simulink model "sensor_test_MIL"  (R2022b)
settings: Solver=FixedStepDiscrete  StartTime=0.0  StopTime=30.0  RelTol=1e-3
InitFcn:
  | mbd_s32k_consistency_checks(bdroot(gcs));
undefined symbols (not defined in the file): LQFP
libraries: mbd_s32k1xx_ec_toolbox x4, hdlsllib x3, aerolibanimutils x1
settings Model: Creator=termi  LastModifiedBy=termi
settings DataIOCC: ExternalInput=off  InitialState=off  SaveOutput=off  SignalLogging=off  SaveTime=off
settings OptimizationCC: DefaultParameterBehavior=Inlined  EnhancedBackFolding=on  PassReuseOutputArgsAs=Individual arguments  ZeroExternalMemoryAtStartup=off  ZeroInternalMemoryAtStartup=off  OptimizeBlockOrder=speed  DifferentSizesBufferReuse=on  OptimizationCustomize=off  EfficientTunableParamExpr=on
settings DebuggingCC: InheritedTsInSrcMsg=none  SingleTaskRateTransMsg=error  ParameterTunabilityLossMsg=error  UnconnectedInputMsg=error  UnconnectedOutputMsg=error  UnconnectedLineMsg=error  UnknownTsInhSupMsg=error
settings HardwareCC: ProdBitPerPointer=32  ProdBitPerSizeT=32  ProdBitPerPtrDiffT=32  ProdLargestAtomicInteger=Long  ProdLargestAtomicFloat=Double  ProdWordSize=32  ProdHWDeviceType=ARM Compatible->ARM Cortex
settings SFSimCC: MATLABDynamicMemAlloc=off
settings RTWCC: Description=Model Based Design Toolbox S32K1xx Code Generation Target  SystemTargetFile=mbd_s32k.tlc  MakeCommand=mbd_s32k_make_rtw COPY_MDLREF_INCLUDES=0  TemplateMakefile=mbd_s32k.tmf
settings CodeAppCC: ForceParamTrailComments=on  IgnoreCustomStorageClasses=off  OperatorAnnotations=on  SimulinkDataObjDesc=on  SFDataObjDesc=on  InsertBlockDesc=on
settings STFCustomTargetCC: TargetLangStandard=C99 (ISO)  MultiwordLength=256  GenerateSampleERTMain=on  CombineOutputUpdateFcns=on  ERTCustomFileBanners=on  SupportContinuousTime=off  SupportNonInlinedSFcns=off  RemoveResetFunc=on  MATLABClassNameForMDSCustomization=Simulink.SoftwareTarget.ERTCustomization  SystemTargetFile=mbd_s32k.tlc
settings ERTTargetCC: TargetLangStandard=C99 (ISO)  GenerateSampleERTMain=on  ParMdlRefBuildCompliant=off  CompOptLevelCompliant=off  ConcurrentExecutionCompliant=off  ModelStepFunctionPrototypeControlCompliant=off  CPPClassGenCompliant=off  UseToolchainInfoCompliant=off  InlinedParameterPlacement=NonHierarchical  ERTSrcFileBannerTemplate=mbd_ert_code_template.cgt  ERTHdrFileBannerTemplate=mbd_ert_code_template.cgt  ERTDataSrcFileTemplate=mbd_ert_code_template.cgt  ERTDataHdrFileTemplate=mbd_ert_code_template.cgt  ERTCustomFileTemplate=example_file_process.tlc

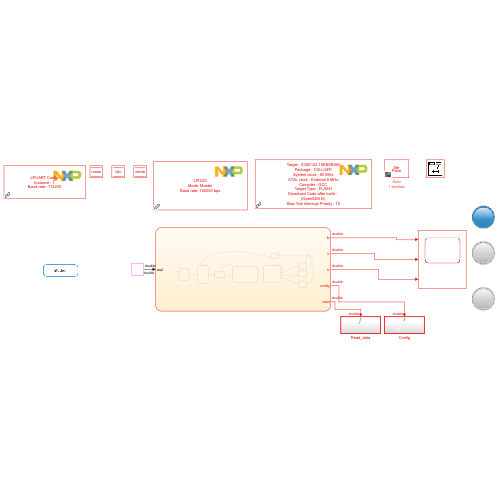
[thumbnail: Simulink's stored preview of the top-level diagram]
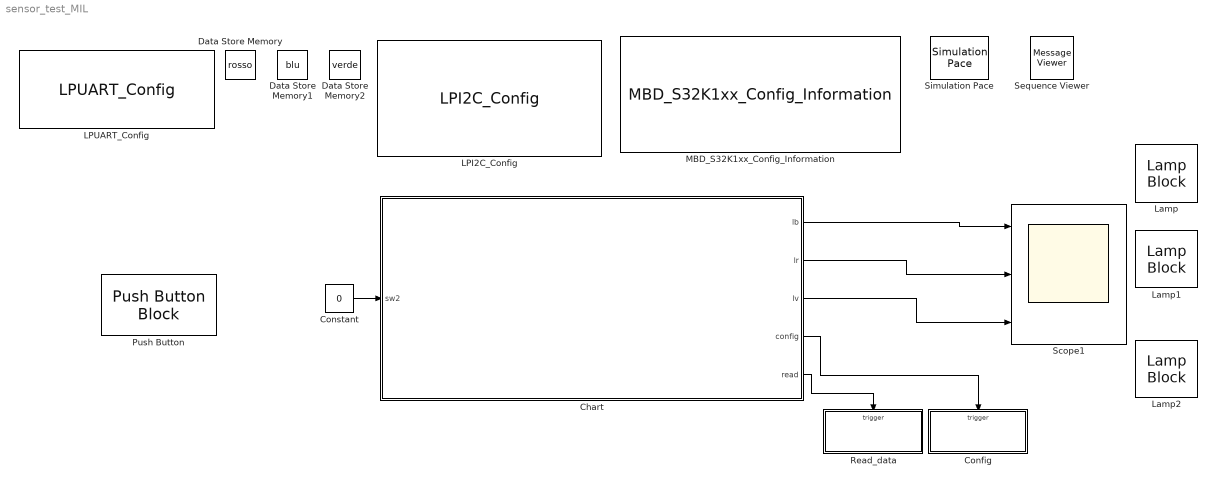
== system sensor_test_MIL ==
  Chart : Stateflow chart  TreatAsAtomicUnit=on
  Config : Subsystem  TreatAsAtomicUnit=on
  Constant : Constant  Value=0
  Data Store Memory : DataStoreMemory  DataStoreName=rosso  WriteAfterWriteMsg=warning  ShowAdditionalParam=off  OutDataTypeStr=uint16
  Data Store Memory1 : DataStoreMemory  DataStoreName=blu  WriteAfterWriteMsg=warning  ShowAdditionalParam=off  OutDataTypeStr=uint16
  Data Store Memory2 : DataStoreMemory  DataStoreName=verde  WriteAfterWriteMsg=warning  ShowAdditionalParam=off  OutDataTypeStr=uint16
  LPI2C_Config : mbd_s32k1xx_ec_toolbox/Communication Blocks/I2C Blocks/LPI2C_Config  Priority=1  instance=0  mode=Master  opmode=Standard (up to 100 kbit/s)  bdr=100000  addr=1  is10bitaddr=off  status=off  sda=PTA2: [LPI2C0_SDA | LPI2C Data I/O]  scl=PTA3: [LPI2C0_SCL | LPI2C Clock I/O]
  LPUART_Config : mbd_s32k1xx_ec_toolbox/Communication Blocks/UART Blocks/LPUART_Config  instance=1  baudrate=115200  custom_baudrate=1000000  databits=8  parity=None  sbns=1  bothedge=rising edge  rxinv=off  txinv=off  show_adv_opts=on  brk13=10 - 13 bit times  lbkde=10 - 13 bit times  rx=PTC6: [LPUART1_RX | Receive]  tx=PTC7: [LPUART1_TX | Transmit]
  Lamp : LampBlock  LabelPosition=Hide
  Lamp1 : LampBlock  LabelPosition=Hide
  Lamp2 : LampBlock  LabelPosition=Hide
  MBD_S32K1xx_Config_Information : mbd_s32k1xx_ec_toolbox/MBD_S32K1xx_Config_Information  Priority=1  mbdt_ver=0  disp_str=|  config_params=[]  mcu_target_name=S32K142  mcu_target_package=100-LQFP  mcu_target_sram_size=16KB  mcu_system_clock_freq=80  mcu_xtal_freq=External 8  mcu_steptick_timer=LPIT Channel 0  mcu_steptick_prio=15  ds_import_enable=on  target_compiler=GCC  target_memory=FLASH  gcc_target_compile_opts=-mthumb -mfloat-abi=hard -mfpu=fpv4-sp-d16 -O1 -g -gstrict-dwarf  gcc_target_assemble_opts=-mthumb -mfloat-abi=hard -mfpu=fpv4-sp-d16 -g  gcc_target_link_opts=-mthumb -mfloat-abi=hard -mfpu=fpv4-sp-d16  gcc_target_default_lcf=on  gcc_target_user_lcf=S32K142_16_flash.ld  ghs_target_compile_opts=-cpu=cortexm4f -thumb -fpu=vfpv4_d16 -fsingle -Ogeneral -Wundef -Wimplicit-int -Wshadow -Wtrigraphs --no_commons --gnu_asm -gnu99 -gdwarf-2 -G  ghs_target_assemble_opts=-cpu=cortexm4f -fpu=vfpv4_d16  ghs_target_link_opts=-cpu=cortexm4f -thumb -fpu=vfpv4_d16  ghs_target_default_lcf=on  ghs_target_user_lcf=S32K142_16_flash.ld  iar_target_compile_opts=--cpu=Cortex-M4F --thumb --fpu=VFPv4_sp -Ol -e --debug --dlib_config normal  iar_target_assemble_opts=--cpu Cortex-M4F --thumb --fpu VFPv4_sp  iar_target_link_opts=--no_exceptions --vfe --inline  iar_target_default_lcf=on  iar_target_user_lcf=S32K142_16_flash.icf  pil_download_enable=off  rbl_download_enable=on  rbl_start_delay=5000  rbl_download_interface=OpenSDA  rbl_restart_request=off  rbl_com_port=Custom  rbl_com_port_custom=COM3  pil_download_rate=115200  pil_download_rate_custom=115200  pil_opensda_drive=Custom  pil_opensda_drive_custom=D  jtag_interface=OpenSDA Embedded Debug  jlink_default_path=on  jlink_user_path=C:\Program Files\SEGGER\JLink\  pil_uart_instance=1  pil_uart_rx=PTC6: [LPUART1_RX | Receive]  pil_uart_tx=PTC7: [LPUART1_TX | Transmit]  FTM_PWM_PcrCheckEnDis=on  FTM_Input_Edge_Inputs_PcrCheckEnDis=on  FTM_Dual_Edge_Inputs_PcrCheckEnDis=on  FTM_Quadrature_Inputs_PcrCheckEnDis=on  FTM_Hall_Sensor_Inputs_PcrCheckEnDis=on  LPTMR_PcrCheckEnDis=on  PIT_PcrCheckEnDis=on  RTC_PcrCheckEnDis=on  FlexCAN_PcrCheckEnDis=on  LIN_PcrCheckEnDis=on  FlexIO_PcrCheckEnDis=on  LPI2C_PcrCheckEnDis=on  LPSPI_PcrCheckEnDis=on  LPUART_PcrCheckEnDis=on  CMP_PcrCheckEnDis=on  GPIO_OutputPcrCheckEnDis=on  GPIO_InputPcrCheckEnDis=on  SBC_PcrCheckEnDis=on  BMS_PcrCheckEnDis=on  AMMCLIB_PcrCheckEnDis=on  FM_PcrCheckEnDis=on  Profile_PcrCheckEnDis=on  ConfigParams_PcrCheckEnDis=on  ModelRef_PcrCheckEnDis=on  PDB0_PcrCheckEnDis=on  CSEc_PcrCheckEnDis=on  eDMA_PcrCheckEnDis=on  FLASH_PcrCheckEnDis=on  ADC_PcrCheckEnDis=on  WDOG_PcrCheckEnDis=on
      | Target : S32K144-64KB_SRAM
      | Package : 100-pin
      | System clock : 80 MHz
      | XTAL clock : External 8 MHz
      | Compiler : IAR
      | Target Type : FLASH
      | Download Code after build : off
      | Step Tick Interrupt Priority : 15
  Push Button : PushButtonBlock  OffValue=0.000000
  Read_data : Subsystem  TreatAsAtomicUnit=on
  Scope1 : Scope  NumInputPorts=3
  Sequence Viewer : MessageViewer
  Simulation Pace : aerolibanimutils/Simulation Pace  SimulationPace=1  SleepMode=Auto  OutputPaceError=off  SampleTime=1/10
  wires:
  Chart/1(lb) -> Scope1/1
  Chart/4(config) -> Config/Trigger
  Chart/3(lv) -> Scope1/3
  Chart/2(lr) -> Scope1/2
  Chart/5(read) -> Read_data/Trigger
  Constant/1 -> Chart/1(sw2)

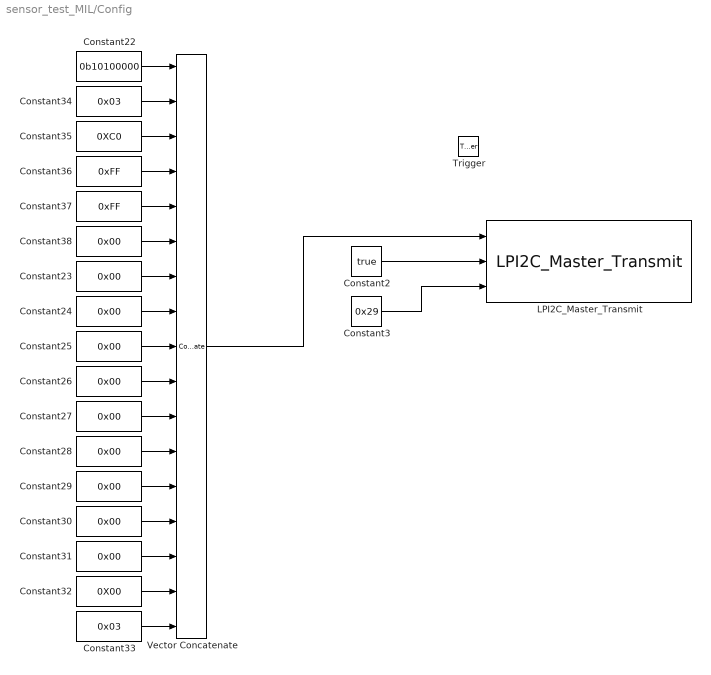
== system sensor_test_MIL/Config ==
  Trigger : TriggerPort  VariantControl=(inherit)  PortDimensions=1
  Constant2 : Constant  Value=true  OutDataTypeStr=boolean
  Constant22 : Constant  Value=0b10100000
  Constant{23..31,38} (10 alike) : Constant  Value=0x00
  Constant3 : Constant  Value=0x29  OutDataTypeStr=uint16
  Constant32 : Constant  Value=0X00
  Constant33 : Constant  Value=0x03
  Constant34 : Constant  Value=0x03
  Constant35 : Constant  Value=0XC0
  Constant36 : Constant  Value=0xFF
  Constant37 : Constant  Value=0xFF
  LPI2C_Master_Transmit : mbd_s32k1xx_ec_toolbox/Communication Blocks/I2C Blocks/LPI2C_Master_Transmit  Priority=1  instance=0  xfermode=Blocking  Timeout=710  is10bit=off  status=off
  Vector Concatenate : Concatenate  NumInputs=17
  wires:
  Constant27/1 -> Vector Concatenate/11
  Constant31/1 -> Vector Concatenate/15
  Constant33/1 -> Vector Concatenate/17
  Constant32/1 -> Vector Concatenate/16
  Constant30/1 -> Vector Concatenate/14
  Vector Concatenate/1 -> LPI2C_Master_Transmit/1
  Constant23/1 -> Vector Concatenate/7
  Constant28/1 -> Vector Concatenate/12
  Constant29/1 -> Vector Concatenate/13
  Constant3/1 -> LPI2C_Master_Transmit/3
  Constant36/1 -> Vector Concatenate/4
  Constant34/1 -> Vector Concatenate/2
  Constant24/1 -> Vector Concatenate/8
  Constant35/1 -> Vector Concatenate/3
  Constant26/1 -> Vector Concatenate/10
  Constant38/1 -> Vector Concatenate/6
  Constant25/1 -> Vector Concatenate/9
  Constant37/1 -> Vector Concatenate/5
  Constant2/1 -> LPI2C_Master_Transmit/2
  Constant22/1 -> Vector Concatenate/1

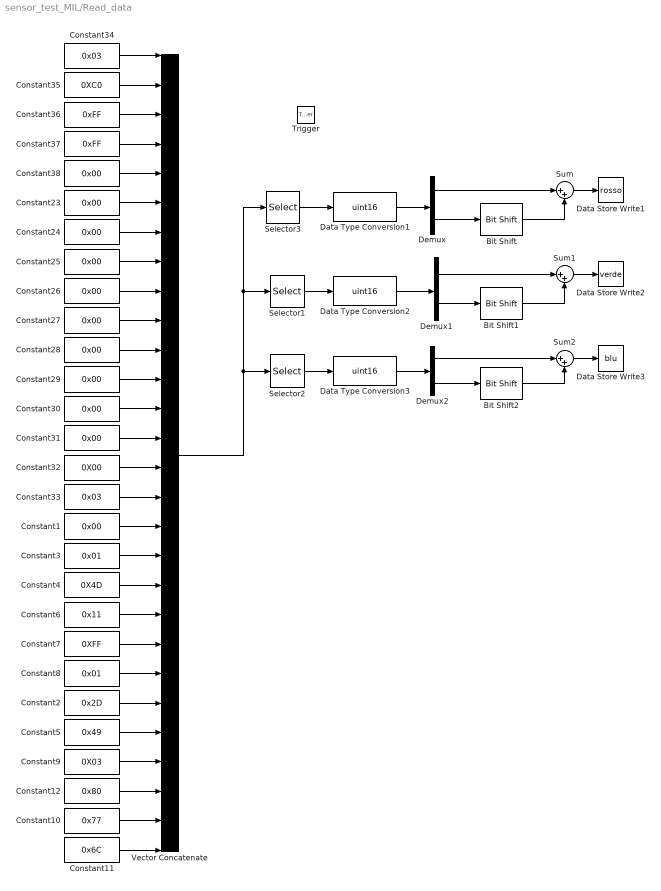
== system sensor_test_MIL/Read_data ==
  Trigger : TriggerPort  VariantControl=(inherit)  PortDimensions=1
  Bit Shift : hdlsllib/Logic and Bit Operations/Bit Shift  mode=Shift Left Logical  N=8
  Bit Shift1 : hdlsllib/Logic and Bit Operations/Bit Shift  mode=Shift Left Logical  N=8
  Bit Shift2 : hdlsllib/Logic and Bit Operations/Bit Shift  mode=Shift Left Logical  N=8
  Constant{1,23..31,38} (11 alike) : Constant  Value=0x00
  Constant10 : Constant  Value=0x77
  Constant11 : Constant  Value=0x6C
  Constant12 : Constant  Value=0x80
  Constant2 : Constant  Value=0x2D
  Constant3 : Constant  Value=0x01
  Constant32 : Constant  Value=0X00
  Constant33 : Constant  Value=0x03
  Constant34 : Constant  Value=0x03
  Constant35 : Constant  Value=0XC0
  Constant36 : Constant  Value=0xFF
  Constant37 : Constant  Value=0xFF
  Constant4 : Constant  Value=0X4D
  Constant5 : Constant  Value=0x49
  Constant6 : Constant  Value=0x11
  Constant7 : Constant  Value=0XFF
  Constant8 : Constant  Value=0x01
  Constant9 : Constant  Value=0X03
  Data Store Write1 : DataStoreWrite  DataStoreName=rosso  IndexOptions=Index vector (dialog)  Indices=1  OutputSizes=1
  Data Store Write2 : DataStoreWrite  DataStoreName=verde  IndexOptions=Index vector (dialog)  Indices=1  OutputSizes=1
  Data Store Write3 : DataStoreWrite  DataStoreName=blu  IndexOptions=Index vector (dialog)  Indices=1  OutputSizes=1
  Data Type Conversion1 : DataTypeConversion  OutDataTypeStr=uint16  SaturateOnIntegerOverflow=off  RndMeth=Floor
  Data Type Conversion2 : DataTypeConversion  OutDataTypeStr=uint16  SaturateOnIntegerOverflow=off  RndMeth=Floor
  Data Type Conversion3 : DataTypeConversion  OutDataTypeStr=uint16  SaturateOnIntegerOverflow=off  RndMeth=Floor
  Demux : Demux  Outputs=2
  Demux1 : Demux  Outputs=2
  Demux2 : Demux  Outputs=2
  Selector1 : Selector  InputPortWidth=28  IndexOptions=Index vector (dialog)  Indices=[25, 26]  OutputSizes=2
  Selector2 : Selector  InputPortWidth=28  IndexOptions=Index vector (dialog)  Indices=[27,28]  OutputSizes=2
  Selector3 : Selector  InputPortWidth=28  IndexOptions=Index vector (dialog)  Indices=[23, 24]  OutputSizes=1
  Sum : Sum  Inputs=|++
  Sum1 : Sum  Inputs=|++
  Sum2 : Sum  Inputs=|++
  Vector Concatenate : Concatenate  NumInputs=28
  wires:
  Vector Concatenate/1 -> Selector3/1, Selector1/1, Selector2/1
  Sum/1 -> Data Store Write1/1
  Selector3/1 -> Data Type Conversion1/1
  Selector1/1 -> Data Type Conversion2/1
  Selector2/1 -> Data Type Conversion3/1
  Data Type Conversion1/1 -> Demux/1
  Sum1/1 -> Data Store Write2/1
  Data Type Conversion2/1 -> Demux1/1
  Sum2/1 -> Data Store Write3/1
  Data Type Conversion3/1 -> Demux2/1
  Demux2/2 -> Bit Shift2/1
  Bit Shift2/1 -> Sum2/2
  Demux1/2 -> Bit Shift1/1
  Bit Shift1/1 -> Sum1/2
  Demux1/1 -> Sum1/1
  Demux/2 -> Bit Shift/1
  Bit Shift/1 -> Sum/2
  Demux/1 -> Sum/1
  Demux2/1 -> Sum2/1
  Constant38/1 -> Vector Concatenate/5
  Constant25/1 -> Vector Concatenate/8
  Constant37/1 -> Vector Concatenate/4
  Constant26/1 -> Vector Concatenate/9
  Constant23/1 -> Vector Concatenate/6
  Constant27/1 -> Vector Concatenate/10
  Constant32/1 -> Vector Concatenate/15
  Constant35/1 -> Vector Concatenate/2
  Constant30/1 -> Vector Concatenate/13
  Constant33/1 -> Vector Concatenate/16
  Constant34/1 -> Vector Concatenate/1
  Constant29/1 -> Vector Concatenate/12
  Constant36/1 -> Vector Concatenate/3
  Constant28/1 -> Vector Concatenate/11
  Constant24/1 -> Vector Concatenate/7
  Constant31/1 -> Vector Concatenate/14
  Constant1/1 -> Vector Concatenate/17
  Constant3/1 -> Vector Concatenate/18
  Constant4/1 -> Vector Concatenate/19
  Constant6/1 -> Vector Concatenate/20
  Constant7/1 -> Vector Concatenate/21
  Constant8/1 -> Vector Concatenate/22
  Constant2/1 -> Vector Concatenate/23
  Constant5/1 -> Vector Concatenate/24
  Constant9/1 -> Vector Concatenate/25
  Constant12/1 -> Vector Concatenate/26
  Constant10/1 -> Vector Concatenate/27
  Constant11/1 -> Vector Concatenate/28

== stateflow chart sensor_test_MIL/Chart ==
  state Time_counter
    en:
    t = t +1;
  state blu_On
    en:
    lb  = 1;
  state wait
    en:
    lb = 0;
    lv = 0;
    lr = 0;
    t = 0;
    i = 1;
    j = 1;
    blu_counter = 0;
    green_counter = 0;
    red_counter = 0;
    config = 0;
  state Voter
    en:
    if( sensing(j) == 1)
    blu_counter = blu_counter +1;
    end
    if( sensing(j) == 2)
    red_counter = red_counter +1;
    end
    if( sensing(j) == 3)
    green_counter = green_counter +1;
    end
    j = j +1;
  state Color_detection
    en:
    read = 0;
    switch true
    case blu > rosso && blu < verde
    sensing(i) = 1;
    case rosso > blu && rosso > verde
    sensing(i) = 2;
    case verde > rosso && verde > blu && blu < rosso
    sensing(i) = 3
    end
    i = i + 1;
  state Sensor_init
    en:
    config = 1;
    read = 0;
  state rosso_on
    en:
    lr  = 1;
  state Sensor_read
    en:
    read = 1;
  state verde_on
    en:
    lv  = 1;
  Time_counter -> wait [order 1] : [t == 25]
  Time_counter -> Time_counter [order 2] : [after(200, msec)]
  verde_on -> (junction 15)
  (junction 15) -> Time_counter
  rosso_on -> (junction 15)
  blu_On -> (junction 15)
  Voter -> Voter [order 4]
  Color_detection -> Sensor_read [order 2] : [after (200, msec)]
  Voter -> blu_On [order 1] : [blu_counter ==2]
  (default) -> Sensor_init
  Sensor_init -> wait : [after (150,msec)]
  wait -> Sensor_read : [sw2 == true]
  Color_detection -> Voter [order 1] : [i == 4]
  Sensor_read -> Color_detection
  Voter -> rosso_on [order 3] : [red_counter == 2]
  Voter -> verde_on [order 2] : [green_counter == 2]
  data: lb output; lr output; lv output; sensing local size=[1, 3] =[0 0 0]; t local; blu_counter local; green_counter local; i local; red_counter local; rosso data_store_memory; verde data_store_memory; config output; blu data_store_memory; j local; read output; sw2 input
